simulink model "TTT_BEMT"  (R2024b)
settings: Solver=VariableStepAuto  StartTime=0.0  StopTime=100  FixedStep=0.01  RelTol=1e-3
settings Model: ExtModeTrigDuration=100  Creator=thogan1  LastModifiedBy=thogan1

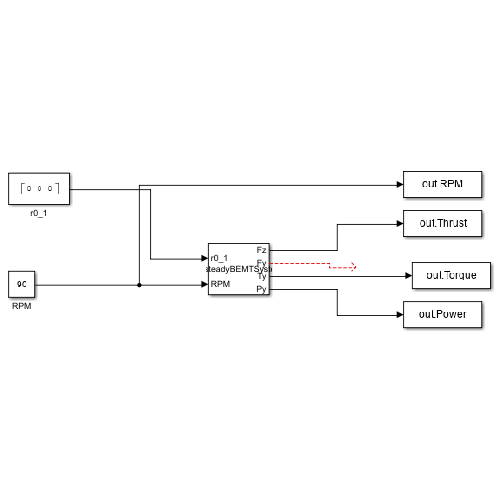
[thumbnail: Simulink's stored preview of the top-level diagram]
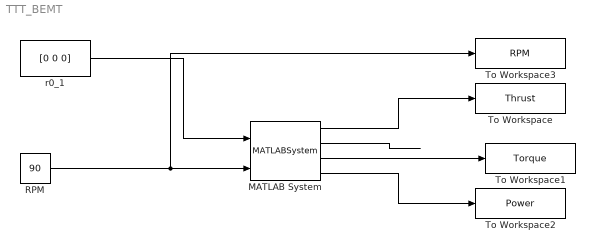
== system TTT_BEMT ==
  MATLAB System : MATLABSystem  System=unsteadyBEMTSystem  dt=0.01  rho=1000  kinVisc=1.004*10^-6  windSpeed_nom=1.4  hhub_nom=4  alphaPowerLaw=1 / 5  betaBedRoughness=1  a=2  towerShadow=false  yaw=0  tilt=0  cone=5  prandtlCorrection=true  prandtlTipLoss=true  prandtlHubLoss=true  glauertCorrection=true  dynamicStall=false  dynamicWake=true  skewedWake=false  ac=1 / 3  Rr=0.75  Rh=0.0035  Rb=[0.72656 0.67969 0.63281 0.58594 0.53906 0.49219 0.44531 0.39844 0.35156 0.30469 0.25781 0.21094 0.16406 0.11719 0.07031 0.02344]  chord=[0.07420 0.08450 0.09454 0.11637 0.12260 0.12703 0.13016 0.13233 0.13380 0.13491 0.13570 0.13640 0.13717 0.13952 0.14050 0.14250]  twist=[83.90487 83.53000 83.39358 82.89349 82.82024 82.65112 82.32417 81.88798 81.36263 80.63447 79.64462 78.37823 76.77522 72.14122 72.00560 71.56956]  pitch=0  nB=3  n=[ 0, 0, -1 ]  linThresh=0.85  polarData=load( 'polarData.mat', 'polarData' )  nDoF=3  SimulateUsing=Code generation
      mask Type: unsteadyBEMTSystem
      mask Display:
      | disp('unsteadyBEMTSystem');
      | port_label('input',1,'r0_1');
      | port_label('input',2,'RPM');
      | port_label('output',1,'Fz');
      | port_label('output',2,'Fy');
      | port_label('output',3,'Ty');
      | port_label('output',4,'Py');
  RPM : Constant  Value=90
  To Workspace : ToWorkspace  VariableName=Thrust  SampleTime=-1
      settings: Save2DSignal=2-D array (concatenate along first dimension)
  To Workspace1 : ToWorkspace  VariableName=Torque  SampleTime=-1
      settings: Save2DSignal=2-D array (concatenate along first dimension)
  To Workspace2 : ToWorkspace  VariableName=Power  SampleTime=-1
      settings: Save2DSignal=2-D array (concatenate along first dimension)
  To Workspace3 : ToWorkspace  VariableName=RPM  SampleTime=-1
      settings: Save2DSignal=2-D array (concatenate along first dimension)
  r0_1 : Constant  Value=[0 0 0]
  wires:
  r0_1/1 -> MATLAB System/1
  RPM/1 -> To Workspace3/1, MATLAB System/2
  MATLAB System/1 -> To Workspace/1
  MATLAB System/2 -> ?
  MATLAB System/3 -> To Workspace1/1
  MATLAB System/4 -> To Workspace2/1
